simulink model "gyro_noise_filter_test"  (R2015b)
settings: Solver=FixedStepDiscrete  StartTime=0.0  StopTime=10.0  FixedStep=sample_test_time  RelTol=1e-3
values from neighbouring files (symbols this model uses):
  sample_test_time = 1/2000    (= 0.0005)    [imu_noise_and_filter_inputs.m]
libraries: util_common_lib x3, util_tf_lib x3
settings Model: Creator=jimkaidy  LastModifiedBy=jimkaidy

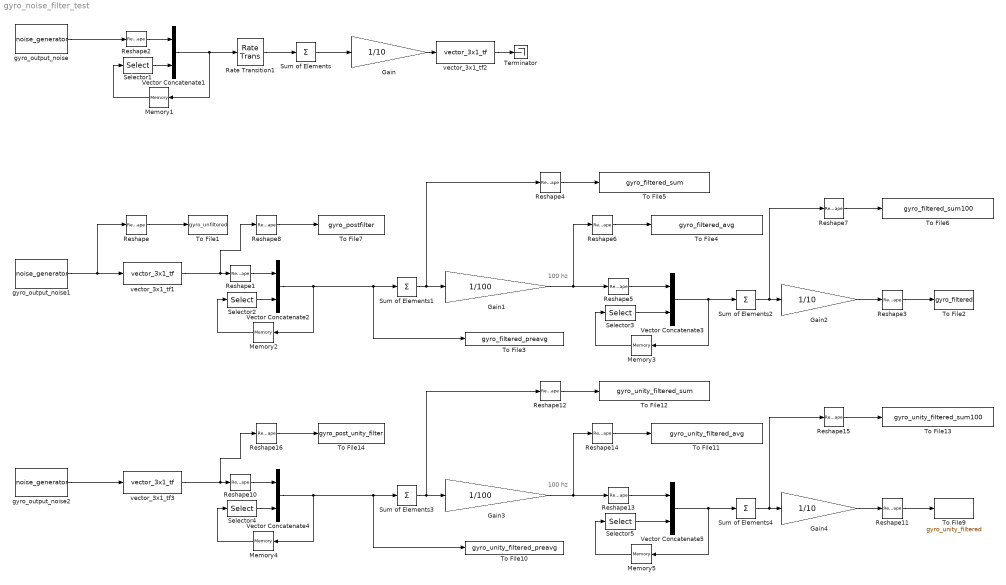
== system gyro_noise_filter_test ==
  note: 100 hz
  note: 100 hz
  Gain : Gain  Gain=1/10
  Gain1 : Gain  Gain=1/100
  Gain2 : Gain  Gain=1/10
  Gain3 : Gain  Gain=1/100
  Gain4 : Gain  Gain=1/10
  Memory1 : Memory  X0=zeros(10,3)  InheritSampleTime=on
  Memory2 : Memory  X0=zeros(1/(sample_test_time*100),3)  InheritSampleTime=on
  Memory3 : Memory  X0=zeros(10,3)  InheritSampleTime=on
  Memory4 : Memory  X0=zeros(1/(sample_test_time*100),3)  InheritSampleTime=on
  Memory5 : Memory  X0=zeros(10,3)  InheritSampleTime=on
  Rate Transition1 : RateTransition
  Reshape{,3..4,6..8,11..12,14..16} (11 alike) : Reshape
  Reshape{1..2,5,10,13} (5 alike) : Reshape  OutputDimensionality=Row vector (2-D)
  Selector1 : Selector  NumberOfDimensions=2  InputPortWidth=10  IndexOptions=Index vector (dialog),Select all  Indices=[1:9],1  OutputSizes=1,1
  Selector2 : Selector  NumberOfDimensions=2  InputPortWidth=10  IndexOptions=Index vector (dialog),Select all  Indices=[1:1/(sample_test_time*100)-1],1  OutputSizes=1,1
  Selector3 : Selector  NumberOfDimensions=2  InputPortWidth=10  IndexOptions=Index vector (dialog),Select all  Indices=[1:9],1  OutputSizes=1,1
  Selector4 : Selector  NumberOfDimensions=2  InputPortWidth=10  IndexOptions=Index vector (dialog),Select all  Indices=[1:1/(sample_test_time*100)-1],1  OutputSizes=1,1
  Selector5 : Selector  NumberOfDimensions=2  InputPortWidth=10  IndexOptions=Index vector (dialog),Select all  Indices=[1:9],1  OutputSizes=1,1
  Sum of Elements{,1..4} (5 alike) : Sum  Inputs=+  CollapseMode=Specified dimension
  Terminator : Terminator
  To File1 : ToFile  Filename=gyro_unfiltered  MatrixName=gyro_unfiltered  SaveFormat=Timeseries
  To File10 : ToFile  Filename=gyro_unity_filtered_preavg  MatrixName=gyro_unity_filtered_preavg  SaveFormat=Timeseries
  To File11 : ToFile  Filename=gyro_unity_filtered_avg  MatrixName=gyro_unity_filtered_avg  SaveFormat=Timeseries
  To File12 : ToFile  Filename=gyro_unity_filtered_sum  MatrixName=gyro_unity_filtered_sum  SaveFormat=Timeseries
  To File13 : ToFile  Filename=gyro_unity_filtered_sum100  MatrixName=gyro_unity_filtered_sum100  SaveFormat=Timeseries
  To File14 : ToFile  Filename=gyro_post_unity_filter  MatrixName=gyro_post_unity_filter  SaveFormat=Timeseries
  To File2 : ToFile  Filename=gyro_filtered  MatrixName=gyro_filtered  SaveFormat=Timeseries
  To File3 : ToFile  Filename=gyro_filtered_preavg  MatrixName=gyro_filtered_preavg  SaveFormat=Timeseries
  To File4 : ToFile  Filename=gyro_filtered_avg  MatrixName=gyro_filtered_avg  SaveFormat=Timeseries
  To File5 : ToFile  Filename=gyro_filtered_sum  MatrixName=gyro_filtered_sum  SaveFormat=Timeseries
  To File6 : ToFile  Filename=gyro_filtered_sum100  MatrixName=gyro_filtered_sum100  SaveFormat=Timeseries
  To File7 : ToFile  Filename=gyro_postfilter  MatrixName=gyro_postfilter  SaveFormat=Timeseries
  To File9 : ToFile  Filename=gyro_unity_filtered  MatrixName=gyro_unity_filtered  SaveFormat=Timeseries
  Vector Concatenate{1..5} (5 alike) : Concatenate  Mode=Multidimensional array
  gyro_output_noise : util_common_lib/noise_generator  std_dev=mhn_gyro_noise_v  bias=mhn_gyro_bias_v  seed=mhn_gyro_seed_v  on=mhn_gyro_noise_on  sample_time=sample_test_time
  gyro_output_noise1 : util_common_lib/noise_generator  std_dev=mhn_gyro_noise_v  bias=mhn_gyro_bias_v  seed=mhn_gyro_seed_v  on=mhn_gyro_noise_on  sample_time=sample_test_time
  gyro_output_noise2 : util_common_lib/noise_generator  std_dev=mhn_gyro_noise_v  bias=mhn_gyro_bias_v  seed=mhn_gyro_seed_v  on=mhn_gyro_noise_on  sample_time=sample_test_time
  vector_3x1_tf1 : util_tf_lib/vector_3x1_tf  num=imh_accel_response_num  den=imh_accel_response_den  st=sample_test_time
  vector_3x1_tf2 : util_tf_lib/vector_3x1_tf  num=imh_accel_response_num  den=imh_accel_response_den  st=sample_test_time*20
  vector_3x1_tf3 : util_tf_lib/vector_3x1_tf  num=1  den=1  st=sample_test_time
  wires:
  vector_3x1_tf2/1 -> Terminator/1
  Vector Concatenate1/1 -> Rate Transition1/1, Memory1/1
  gyro_output_noise/1 -> Reshape2/1
  Sum of Elements/1 -> Gain/1
  Selector1/1 -> Vector Concatenate1/2
  Memory1/1 -> Selector1/1
  Gain/1 -> vector_3x1_tf2/1
  Rate Transition1/1 -> Sum of Elements/1
  Reshape2/1 -> Vector Concatenate1/1
  gyro_output_noise1/1 -> Reshape/1, vector_3x1_tf1/1
  vector_3x1_tf1/1 -> Reshape8/1, Reshape1/1
  Selector2/1 -> Vector Concatenate2/2
  Memory2/1 -> Selector2/1
  Reshape1/1 -> Vector Concatenate2/1
  Sum of Elements1/1 -> Reshape4/1, Gain1/1
  Reshape/1 -> To File1/1
  Reshape3/1 -> To File2/1
  Vector Concatenate3/1 -> Sum of Elements2/1, Memory3/1
  Selector3/1 -> Vector Concatenate3/2
  Memory3/1 -> Selector3/1
  Reshape5/1 -> Vector Concatenate3/1
  Gain1/1 -> Reshape6/1, Reshape5/1
  Reshape6/1 -> To File4/1
  Gain2/1 -> Reshape3/1
  Vector Concatenate2/1 -> Sum of Elements1/1, To File3/1, Memory2/1
  Reshape4/1 -> To File5/1
  Sum of Elements2/1 -> Reshape7/1, Gain2/1
  Reshape7/1 -> To File6/1
  Reshape8/1 -> To File7/1
  gyro_output_noise2/1 -> vector_3x1_tf3/1
  vector_3x1_tf3/1 -> Reshape10/1, Reshape16/1
  Selector4/1 -> Vector Concatenate4/2
  Memory4/1 -> Selector4/1
  Reshape10/1 -> Vector Concatenate4/1
  Sum of Elements3/1 -> Gain3/1, Reshape12/1
  Reshape11/1 -> To File9/1
  Vector Concatenate5/1 -> Memory5/1, Sum of Elements4/1
  Selector5/1 -> Vector Concatenate5/2
  Memory5/1 -> Selector5/1
  Reshape13/1 -> Vector Concatenate5/1
  Gain3/1 -> Reshape13/1, Reshape14/1
  Reshape14/1 -> To File11/1
  Gain4/1 -> Reshape11/1
  Vector Concatenate4/1 -> Memory4/1, To File10/1, Sum of Elements3/1
  Reshape12/1 -> To File12/1
  Sum of Elements4/1 -> Gain4/1, Reshape15/1
  Reshape15/1 -> To File13/1
  Reshape16/1 -> To File14/1
